simulink model "QuaternionKinematics"  (Simulink 10.3)
settings: Solver=ode5  StartTime=0.0  StopTime=300  FixedStep=0.01  RelTol=1e-3
libraries: aerosimlib x2, uavutilslib x1
settings Model: Creator=SuturinDA  LastModifiedBy=PC
settings SolverCC: AlgebraicLoopSolver=Auto
settings DataIOCC: SaveFormat=Dataset  SignalLoggingSaveFormat=Dataset  ReturnWorkspaceOutputs=on
settings OptimizationCC: ExpressionDepthLimit=128  LifeSpan=auto
settings DebuggingCC: UnderspecifiedInitializationDetection=Simplified  MergeDetectMultiDrivingBlocksExec=error  FcnCallInpInsideContextMsg=error  StateNameClashWarn=none  SFUnexpectedBacktrackingDiag=error  SFNoUnconditionalDefaultTransitionDiag=error  SFExecutionAtInitializationDiag=warning  SFMachineParentedDataDiag=error  ArithmeticOperatorsInVariantConditions=error
settings HardwareCC: ProdBitPerPointer=64  ProdBitPerSizeT=64  ProdBitPerPtrDiffT=64  ProdLargestAtomicFloat=Float  ProdIntDivRoundTo=Zero  ProdEndianess=LittleEndian  ProdWordSize=64  ProdHWDeviceType=Intel->x86-64 (Windows64)
settings ModelReferenceCC: PropagateSignalLabelsOutOfModel=on
settings SFSimCC: SimUseLocalCustomCode=on  CustomCodeUndefinedFunction=FilterOut
settings RTWCC: RTWUseLocalCustomCode=on
settings CodeAppCC: StateflowObjectComments=off
settings GRTTargetCC: TargetLangStandard=C99 (ISO)  CombineOutputUpdateFcns=on  GRTInterface=off
settings ConfigComp: CovMetricSettings=dwe  CovSaveCumulativeToWorkspaceVar=off  CovSaveSingleToWorkspaceVar=off  CovExternalEMLEnable=on

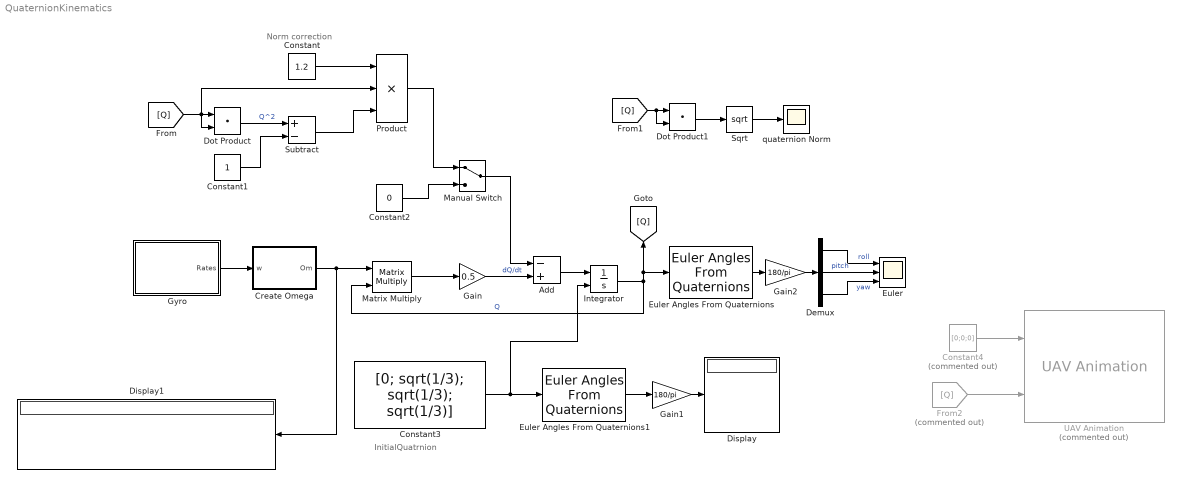
== system QuaternionKinematics ==
  note: Norm correction
  note: InitialQuatrnion
  Add : Sum  Inputs=-+
  Constant : Constant  Value=1.2
  Constant1 : Constant
  Constant2 : Constant  Value=0
  Constant3 : Constant  Value=[0; sqrt(1/3); sqrt(1/3); sqrt(1/3)]
  Constant4 : Constant  Commented=on  Value=[0;0;0]
  Create Omega : MATLAB Function  TreatAsAtomicUnit=on
  Demux : Demux  Outputs=3
  Display : Display
  Display1 : Display
  Dot Product : DotProduct  InputSameDT=on  OutDataTypeStr=Inherit: Inherit via internal rule
  Dot Product1 : DotProduct  InputSameDT=on  OutDataTypeStr=Inherit: Inherit via internal rule
  Euler : Scope  NumInputPorts=3
  Euler Angles From Quaternions : aerosimlib/Transformations/Euler Angles From Quaternions
  Euler Angles From Quaternions1 : aerosimlib/Transformations/Euler Angles From Quaternions
  From2 : From  Commented=on  GotoTag=Q
  Gain : Gain  Gain=0.5
  Gain1 : Gain  Gain=180/pi
  Gain2 : Gain  Gain=180/pi
  Gyro : Subsystem
  Integrator : Integrator  InitialConditionSource=external  InitialCondition=[0; 0; 0; 1]
  Manual Switch : ManualSwitch
  Matrix Multiply : Product  Multiplication=Matrix(*)
  Product : Product  Inputs=3
  Sqrt : Sqrt  SaturateOnIntegerOverflow=on
  Subtract : Sum  Inputs=+-
  UAV Animation : uavutilslib/UAV Animation  Commented=on  UAVType=FixedWing  UAVSize=5  InertialZDirection=Down  SampleTime=-1
      settings: SourceProductBaseCode=UV
  quaternion Norm : Scope
  wires:
  Gyro/1(Rates) -> Create Omega/1(w)
  Create Omega/1(Om) -> Display1/1, Matrix Multiply/1
  Matrix Multiply/1 -> Gain/1
  Gain/1 -> Add/2  "dQ/dt"
  Integrator/1 -> [Q], Euler Angles From Quaternions/1, Matrix Multiply/2  "Q"
  Constant/1 -> Product/1
  Add/1 -> Integrator/1
  Dot Product/1 -> Subtract/1  "Q^2"
  Product/1 -> Manual Switch/1
  Subtract/1 -> Product/3
  Constant1/1 -> Subtract/2
  [Q] -> Dot Product/2, Product/2, Dot Product/1
  Manual Switch/1 -> Add/1
  Constant2/1 -> Manual Switch/2
  Euler Angles From Quaternions/1 -> Gain2/1
  Demux/1 -> Euler/1  "roll"
  Demux/2 -> Euler/2  "pitch"
  Demux/3 -> Euler/3  "yaw"
  Euler Angles From Quaternions1/1 -> Gain1/1
  Constant3/1 -> Euler Angles From Quaternions1/1, Integrator/2
  Gain1/1 -> Display/1
  Gain2/1 -> Demux/1
  [Q] -> Dot Product1/2, Dot Product1/1
  Dot Product1/1 -> Sqrt/1
  Sqrt/1 -> quaternion Norm/1
  Constant4/1 -> UAV Animation/1
  From2/1 -> UAV Animation/2

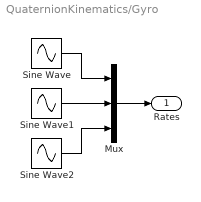
== system QuaternionKinematics/Gyro ==
  Mux : Mux  Inputs=3
  Sine Wave : Sin  Amplitude=5*pi/180  Frequency=10*pi/180  SampleTime=0
  Sine Wave1 : Sin  Amplitude=3*pi/180  Frequency=10*pi/180  SampleTime=0
  Sine Wave2 : Sin  Amplitude=0.5*pi/180  Frequency=10*pi/180  SampleTime=0
  Rates : Outport
  wires:
  Mux/1 -> Rates/1
  Sine Wave/1 -> Mux/1
  Sine Wave1/1 -> Mux/2
  Sine Wave2/1 -> Mux/3

== matlab function Create Omega ==
  data: w input double; Om output double
function Om = fcn(w)
    p = w(1);
    q= w(2);
    r = w(3);

    Om = [[0 -p -q -r];
            [p 0 r q];
            [q -r 0 p];
            [r q -p 0]];
